simulink model "DSPB_MMSE"  (Simulink 8.1)
settings: Solver=VariableStepDiscrete  StartTime=0.0  StopTime=DSPB_MMSE_param.endTime  RelTol=1e-3
PreLoadFcn:
  | % Run the setup script when the model is opened
  | setup_DSPB_MMSE;
InitFcn:
  | % Run the setup script again just before the
  | % model is run, so that any updates made
  | % after opening are applied.
  | setup_DSPB_MMSE;
  | %% DSPBuilder Start
  | alt_dspbuilder_update_model(bdroot)
  | %% DSPBuilder End
StartFcn:
  | %% DSPBuilder Start
  | alt_dspbuilder_hdlimport_prepare_for_simulation(bdroot)
  | %% DSPBuilder End
undefined symbols (not defined in the file or in its folder): a, AdvDSPBDMemDisplay, dpoly, DSPB_MMSE_param, dspba, evalAionMaskParam, pow, primtype, UseDontCare, value, x, y
libraries: DSPBAPrim x213, DspbAdvFftLibrary x9, DSPBABase x5, simulink x3, DSPBAModelBus x3, DSPBAControl x1, DSPBAVectorUtil x1
(part 1 of 3)
Description:
  | DSP Builder Advanced Template for Template Design implementing Primitive Subsystems
settings Model: Creator=mjervis  LastModifiedBy=AliReza
settings DebuggingCC: InheritedTsInSrcMsg=none  IntegerOverflowMsg=none  FcnCallInpInsideContextMsg=EnableAllAsError  FrameProcessingCompatibilityMsg=error
settings GRTTargetCC: CodeReplacementLibrary=None  CPPClassGenCompliant=on

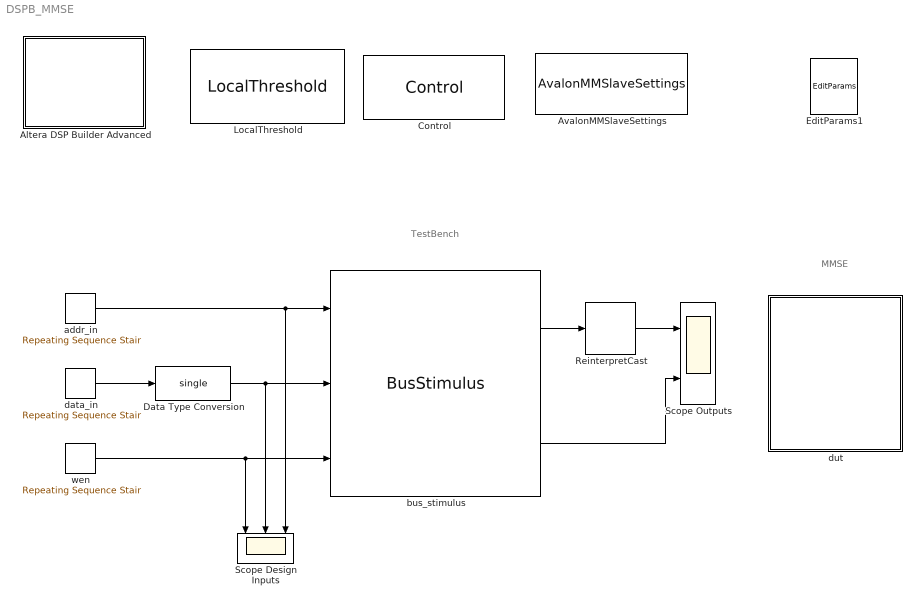
== system DSPB_MMSE ==
  note: MMSE
  note: TestBench
  Altera DSP Builder Advanced : Subsystem  mask(DSP Builder Advanced Blockset Ignored Block){}
      settings: OpenFcn=web('http://www.altera.com', '-new');
      mask Display: image(imread('intellogo.tif'));
  AvalonMMSlaveSettings : DSPBABase/AvalonMMSlaveSettings
  "Control " : DSPBABase/Control  generate=on  language=VHDL  destination=./rtl  make_full_path=off  path_is_relative=on  autotestbench=on  signaldepth=2  coveragetestbench=off  logs=off  spacewidth=2  spacenum=1  addrwidth=10  datawidth=16  dataendian=Big Endian  hierarchicalnames=on  ramThresholdBits=-1  distRamThresholdBits=-1  mlabThresholdBits=-1  hardMultiplierThresholdLuts=-1  version=20090407  errorOnChanMismatch=1  errorOnGPIOMismatch=0  importModelsimResults=0  cycleAccurate=off  reinterpretCastMult=off  paramFile=DSPB_MMSE_params.xml
  Data Type Conversion : DataTypeConversion  OutDataTypeStr=single
  EditParams1 : DSPBABase/EditParams  version=20090407
  LocalThreshold : DSPBABase/LocalThreshold  margin=0  delayRegOrRAMThresholdBits=-1  MediumDualMemThresholdBits=-1  LargeDualMemThresholdBits=0  hardMultiplierThresholdLuts=0  complexMultKaratsuba=off  version=0
  ReinterpretCast : DSPBAPrim/ReinterpretCast  primtype=reinterpret  nInputs=1  nOutputs=1  omode=single  otype=sfix(16)  scale=2^-15  rndmethod=Unbiased  factor=1  satmethod=Symmetric  shift_vec=[0 1 2 -1]  value=0  inPortNames=[' '; ' ';]  outPortNames=[' ']  dspbaimage=dspba_prim.jpg  text=fprintf('Reinterp\nCast', value);  style=Optimised  visibilities=8  floatPrecision=float32_m23  version=20120601
  Scope Outputs : Scope  NumInputPorts=2
      settings: YMin=-5~-5  YMax=5~5
  Scope Design Inputs : Scope  NumInputPorts=3
      settings: YMin=0~-0.05~-5  YMax=1~1~5
  addr_in : simulink/Sources/Repeating Sequence Stair  OutValues=DSPB_MMSE_IO.bus_addr_in  tsamp=1  OutMin=[]  OutMax=[]  OutDataTypeStr=Inherit: Inherit via back propagation  OutDataType=uint10  ConRadixGroup=Best Precision: Vector-wise  OutScaling=[]
  bus_stimulus : DSPBAModelBus/BusStimulus  SampleTime=-1  version=20140122  hasreaden=off
  data_in : simulink/Sources/Repeating Sequence Stair  OutValues=DSPB_MMSE_IO.bus_data_in  tsamp=1  OutMin=[]  OutMax=[]  OutDataTypeStr=double  OutputDataTypeScalingMode=double  OutDataType=fixdt(0,3)  ConRadixGroup=Best Precision: Vector-wise  OutScaling=[]
  dut : Subsystem
  wen : simulink/Sources/Repeating Sequence Stair  OutValues=DSPB_MMSE_IO.bus_wen  tsamp=1  OutMin=[]  OutMax=[]  OutDataTypeStr=fixdt('boolean')  OutputDataTypeScalingMode=Specify via dialog  OutDataType=fixdt('boolean')  ConRadixGroup=Best Precision: Vector-wise  OutScaling=[]
  wires:
  bus_stimulus/2 -> Scope Outputs/2
  addr_in/1 -> Scope Design Inputs/3, bus_stimulus/1
  wen/1 -> Scope Design Inputs/1, bus_stimulus/3
  data_in/1 -> Data Type Conversion/1
  Data Type Conversion/1 -> Scope Design Inputs/2, bus_stimulus/2
  bus_stimulus/1 -> ReinterpretCast/1
  ReinterpretCast/1 -> Scope Outputs/1

== system DSPB_MMSE/Altera DSP Builder Advanced ==

== system DSPB_MMSE/dut ==
  Device : DSPBABase/Device  family=Cyclone V  deviceMember=Stratix V GX  stratix4device=Stratix IV E  hardcopy4device=HardCopy IV E  stratix5device=Stratix V GX  device=AUTO  speed=-3  stratixSpeed=-5  stratix2Speed=-3  stratix3Speed=-2  stratix4gxSpeed=-2  stratix4gtSpeed=-1  cyclone2Speed=-6  cyclone3Speed=-7  arria2Speed=-4  cyclone4eSpeed=-8  stratix5Speed=-3  arria5Speed=-4  arriaSpeed=-6  cyclone3lsSpeed=-7  cyclone5Speed=-6  arria2gzSpeed=-3  nightFurySpeed=-2  ecp2Speed=-7  hardcopycompat=off  version=20140217  max10flashmode=off  max10nomeminit=off
  MMSE_TOP : Subsystem
  MM_in : Subsystem
  MM_out : Subsystem
  wires:
  MM_in/1(time_sample_valid) -> MMSE_TOP/1(valid)
  MM_in/2(time_sample_input) -> MMSE_TOP/2(sample_in)
  MMSE_TOP/1(_valid) -> MM_out/1(valid)
  MMSE_TOP/2(sample_out) -> MM_out/2(time_sample_output)

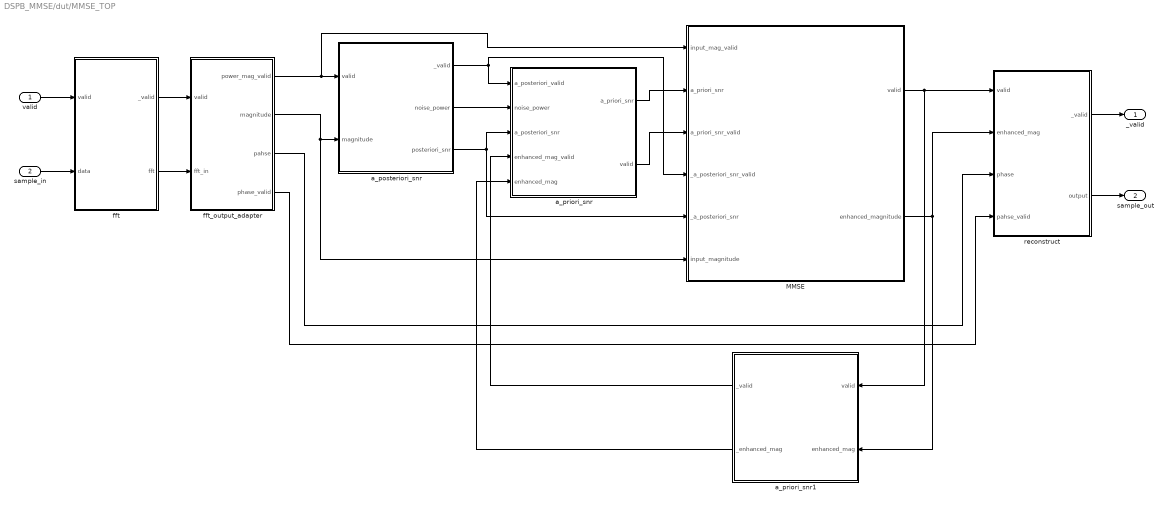
== system DSPB_MMSE/dut/MMSE_TOP ==
  valid : Inport
  sample_in : Inport  Port=2
  MMSE : Subsystem
  a_posteriori_snr : Subsystem
  a_priori_snr : Subsystem
  a_priori_snr1 : Subsystem
  fft : Subsystem
  fft_output_adapter : Subsystem
  reconstruct : Subsystem
  _valid : Outport
  sample_out : Outport  Port=2
  wires:
  fft_output_adapter/2(magnitude) -> MMSE/6(input_magnitude), a_posteriori_snr/2(magnitude)
  fft/1(_valid) -> fft_output_adapter/1(valid)
  fft/2(fft) -> fft_output_adapter/2(fft_in)
  fft_output_adapter/3(pahse) -> reconstruct/3(phase)
  fft_output_adapter/1(power_mag_valid) -> MMSE/1(input_mag_valid), a_posteriori_snr/1(valid)
  valid/1 -> fft/1(valid)
  sample_in/1 -> fft/2(data)
  fft_output_adapter/4(phase_valid) -> reconstruct/4(pahse_valid)
  reconstruct/1(_valid) -> _valid/1
  reconstruct/2(output) -> sample_out/1
  MMSE/1(valid) -> a_priori_snr1/1(valid), reconstruct/1(valid)
  MMSE/2(enhanced_magnitude) -> reconstruct/2(enhanced_mag), a_priori_snr1/2(enhanced_mag)
  a_priori_snr/1(a_priori_snr) -> MMSE/2(a_priori_snr)
  a_posteriori_snr/3(posteriori_snr) -> MMSE/5(_a_posteriori_snr), a_priori_snr/3(a_posteriori_snr)
  a_posteriori_snr/1(_valid) -> MMSE/4(_a_posteriori_snr_valid), a_priori_snr/1(a_posteriori_valid)
  a_posteriori_snr/2(noise_power) -> a_priori_snr/2(noise_power)
  a_priori_snr/2(valid) -> MMSE/3(a_priori_snr_valid)
  a_priori_snr1/2(_enhanced_mag) -> a_priori_snr/5(enhanced_mag)
  a_priori_snr1/1(_valid) -> a_priori_snr/4(enhanced_mag_valid)

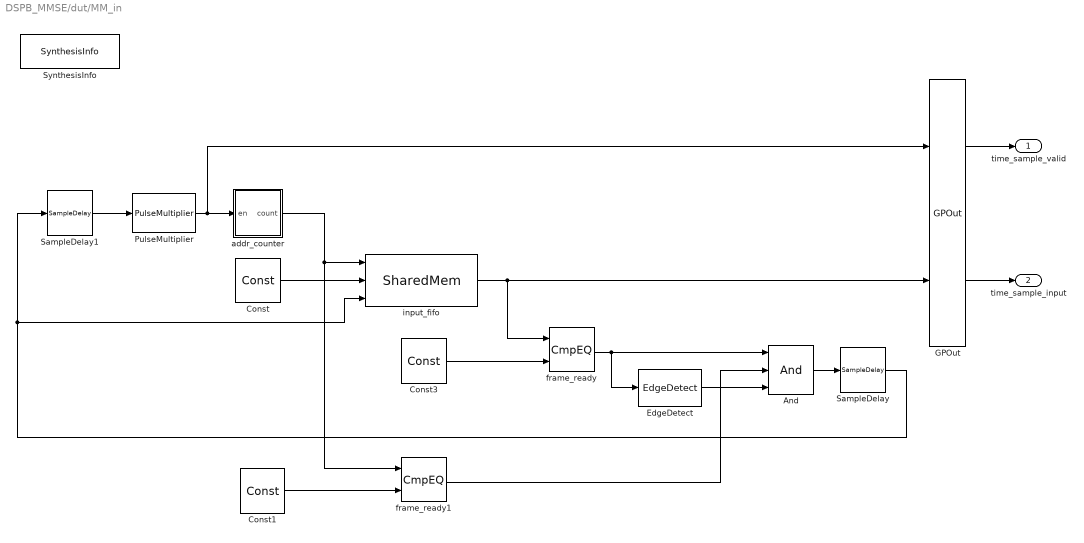
== system DSPB_MMSE/dut/MM_in ==
  And : DSPBAPrim/And  primtype=and  nInputs=3  nOutputs=1  omode=Inherit via internal rule  otype=sfix(16)  scale=2^-15  rndmethod=Unbiased  factor=1  satmethod=Symmetric  shift_vec=[0 1 2 -1]  value=0  inPortNames=[' '; ' '; ' '; ' '; ' '; ' '; ' '; ' '; ' '; ' '; ' '; ' '; ' '; ' '; ' '; ' '; ]  outPortNames=[' ']  dspbaimage=dspba_prim.jpg  text=fprintf('&');  style=Optimised  visibilities=8+2  version=20090407
  Const : DSPBAPrim/Const  primtype=const  nInputs=0  nOutputs=1  omode=single  otype=sfix(16)  scale=2^-15  rndmethod=Unbiased  factor=1  satmethod=Symmetric  shift_vec=[0 1 2 -1]  value=0  inPortNames=['+'; '+';]  outPortNames=[' ']  dspbaimage=dspba_prim.jpg  text=fprintf('%s', num2str(value));  style=Optimised  visibilities=8 + 1024  floatPrecision=float32_m23  version=20120820
  Const1 : DSPBAPrim/Const  primtype=const  nInputs=0  nOutputs=1  omode=Specify via dialog  otype=ufix(DSPB_MMSE_param.FS+1)  scale=2^-0  rndmethod=Unbiased  factor=1  satmethod=Symmetric  shift_vec=[0 1 2 -1]  value=0  inPortNames=['+'; '+';]  outPortNames=[' ']  dspbaimage=dspba_prim.jpg  text=fprintf('%s', num2str(value));  style=Optimised  visibilities=8 + 1024  floatPrecision=float32_m23  version=20120820
  Const3 : DSPBAPrim/Const  primtype=const  nInputs=0  nOutputs=1  omode=single  otype=sfix(16)  scale=2^-15  rndmethod=Unbiased  factor=1  satmethod=Symmetric  shift_vec=[0 1 2 -1]  value=1  inPortNames=['+'; '+';]  outPortNames=[' ']  dspbaimage=dspba_prim.jpg  text=fprintf('%s', num2str(value));  style=Optimised  visibilities=8 + 1024  floatPrecision=float32_m23  version=20120820
  EdgeDetect : DspbAdvFftLibrary/Common/EdgeDetect
  GPOut : DSPBAPrim/GPOut  primtype=gpout  nInputs=evalAionMaskParam(gcb,'value',1)  nOutputs=evalAionMaskParam(gcb,'value',1)  omode=Inherit via internal rule  otype=sfix(16)  scale=2^-15  rndmethod=Unbiased  factor=1  satmethod=Symmetric  shift_vec=[0 1 2 -1]  value=2  inPortNames=[' ' ' ' ' ' ' ' ' ' ' ' ' ' ' ' ' ' ' ' ' ' ' ' ' ' ' ' ' ' ' ' ' ' ' ' ' ' ' ' ' ' ' ' ' ' ' ' ' ' ' ' ' ' ' ' ' ' ' ' ' ' ' ' ' ' ' ' ' ']'  outPortNames=[' ' ' ' ' ' ' ' ' ' ' ' ' ' ' ' ' ' ' ' ' ' ' ' ' ' ' ' ' ' ' ' ' ' ' ' ' ' ' ' ' ' ' ' ' ' ' ' ' ' ' ' ' ' ' ' ' ' ' ' ' ' ' ' ' ' ' ' ' ']'  dspbaimage=dspba_prim.jpg  text=fprintf('GPOut');  style=Optimised  visibilities=1024  latencyCorrection=0  version=20090407
  PulseMultiplier : DspbAdvFftLibrary/Common/PulseMultiplier  N=DSPB_MMSE_param.FS
  SampleDelay : DSPBAPrim/SampleDelay  primtype=sampdelay  nInputs=1  nOutputs=1  omode=Inherit via internal rule  otype=sfix(16)  scale=2^-15  rndmethod=Unbiased  factor=1  satmethod=Symmetric  shift_vec=[0 1 2 -1]  value=3  inPortNames=[' '; ' ';]  outPortNames=[' ']  dspbaimage=dspba_prim.jpg  text=dpoly(1, eye(1,value+1), 'z')  style=Optimised  visibilities=8 + 1024 + 2^17 + 2^18  flexible=off  slackgroup=0  augmented=0  version=20090407  advOptions=[]
  SampleDelay1 : DSPBAPrim/SampleDelay  primtype=sampdelay  nInputs=1  nOutputs=1  omode=Inherit via internal rule  otype=sfix(16)  scale=2^-15  rndmethod=Unbiased  factor=1  satmethod=Symmetric  shift_vec=[0 1 2 -1]  value=1  inPortNames=[' '; ' ';]  outPortNames=[' ']  dspbaimage=dspba_prim.jpg  text=dpoly(1, eye(1,value+1), 'z')  style=Optimised  visibilities=8 + 1024 + 2^17 + 2^18  flexible=off  slackgroup=0  augmented=0  version=20090407  advOptions=[]
  SynthesisInfo : DSPBAPrim/SynthesisInfo  primtype=synthinfo  nInputs=0  nOutputs=0  omode=Inherit via internal rule  otype=sfix(16)  scale=2^-15  rndmethod=Truncate  factor=1  satmethod=Symmetric  shift_vec=[0 1 2 -1]  value=99  inPortNames=[' '; ' ';]  outPortNames=[' ']  dspbaimage=dspba_prim_ctrl.jpg  text=fprintf('Style=%s', style);  style=Scheduled  visibilities=2^17+2^18+2^19+2^20  constraintInUse=off  constraintRelation=>  constraintLimit=2  bitAccurate=off  version=20150220
  addr_counter : Subsystem
  frame_ready : DSPBAPrim/CmpEQ  primtype=cmpeq  nInputs=2  nOutputs=1  omode=boolean  otype=sfix(16)  scale=2^-15  rndmethod=Unbiased  factor=1  satmethod=Symmetric  shift_vec=[0 1 2 -1]  value=0  inPortNames=[' '; ' ';]  outPortNames=[' ']  dspbaimage=dspba_prim.jpg  text=fprintf('==');  style=Optimised  visibilities=0  advOptions=[]  version=20130117
  frame_ready1 : DSPBAPrim/CmpEQ  primtype=cmpeq  nInputs=2  nOutputs=1  omode=boolean  otype=sfix(16)  scale=2^-15  rndmethod=Unbiased  factor=1  satmethod=Symmetric  shift_vec=[0 1 2 -1]  value=0  inPortNames=[' '; ' ';]  outPortNames=[' ']  dspbaimage=dspba_prim.jpg  text=fprintf('==');  style=Optimised  visibilities=0  advOptions=[]  version=20130117
  input_fifo : DSPBAModelBus/SharedMem  mem_addr=0  mem_rwmode=Read/Write  mem_data=zeros(1,2^(DSPB_MMSE_param.FS)+1)  mem_init=on  mem_desc=input fifo  mem_mode=single  mem_type=sfix(16)  mem_scale=2^-8  SampleTime=-1  version=20090407
  time_sample_valid : Outport
  time_sample_input : Outport  Port=2
  wires:
  Const3/1 -> frame_ready/2
  And/1 -> SampleDelay/1
  SampleDelay/1 -> SampleDelay1/1, input_fifo/3
  addr_counter/1(count) -> input_fifo/1, frame_ready1/1
  SampleDelay1/1 -> PulseMultiplier/1
  frame_ready/1 -> EdgeDetect/1, And/1
  frame_ready1/1 -> And/2
  Const1/1 -> frame_ready1/2
  PulseMultiplier/1 -> GPOut/1, addr_counter/1(en)
  GPOut/2 -> time_sample_input/1
  EdgeDetect/1 -> And/3
  input_fifo/1 -> GPOut/2, frame_ready/1
  GPOut/1 -> time_sample_valid/1
  Const/1 -> input_fifo/2

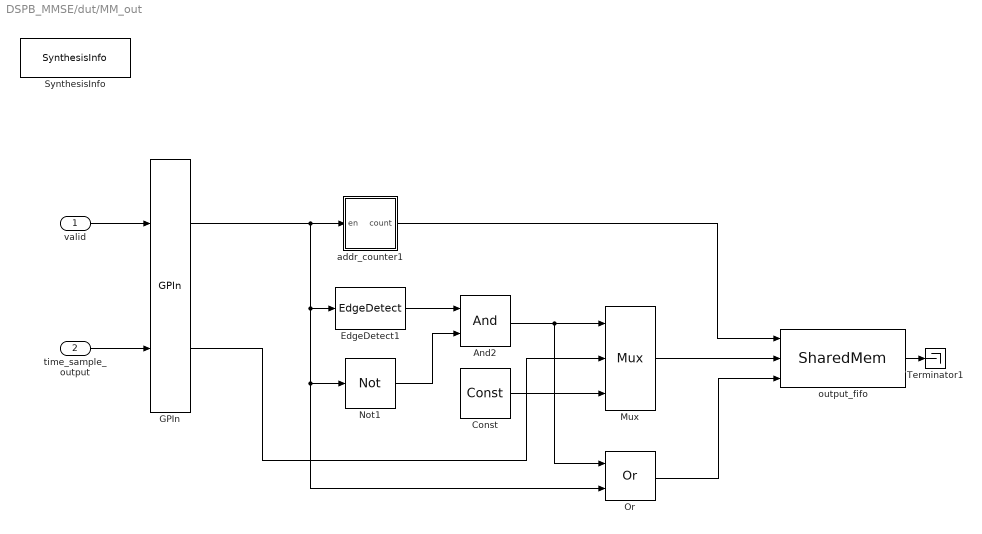
== system DSPB_MMSE/dut/MM_out ==
  valid : Inport
  time_sample_output : Inport  Port=2
  And2 : DSPBAPrim/And  primtype=and  nInputs=2  nOutputs=1  omode=Inherit via internal rule  otype=sfix(16)  scale=2^-15  rndmethod=Unbiased  factor=1  satmethod=Symmetric  shift_vec=[0 1 2 -1]  value=0  inPortNames=[' '; ' '; ' '; ' '; ' '; ' '; ' '; ' '; ' '; ' '; ' '; ' '; ' '; ' '; ' '; ' '; ]  outPortNames=[' ']  dspbaimage=dspba_prim.jpg  text=fprintf('&');  style=Optimised  visibilities=8+2  version=20090407
  Const : DSPBAPrim/Const  primtype=const  nInputs=0  nOutputs=1  omode=single  otype=sfix(16)  scale=2^-15  rndmethod=Unbiased  factor=1  satmethod=Symmetric  shift_vec=[0 1 2 -1]  value=1  inPortNames=['+'; '+';]  outPortNames=[' ']  dspbaimage=dspba_prim.jpg  text=fprintf('%s', num2str(value));  style=Optimised  visibilities=8 + 1024  floatPrecision=float32_m23  version=20120820
  EdgeDetect1 : DspbAdvFftLibrary/Common/EdgeDetect
  GPIn : DSPBAPrim/GPIn  primtype=gpin  nInputs=evalAionMaskParam(gcb,'value',1)  nOutputs=evalAionMaskParam(gcb,'value',1)  omode=Inherit via internal rule  otype=sfix(16)  scale=2^-15  rndmethod=Unbiased  factor=1  satmethod=Symmetric  shift_vec=[0 1 2 -1]  value=2  inPortNames=[' ' ' ' ' ' ' ' ' ' ' ' ' ' ' ' ' ' ' ' ' ' ' ' ' ' ' ' ' ' ' ' ' ' ' ' ' ' ' ' ' ' ' ' ' ' ' ' ' ' ' ' ' ' ' ' ' ' ' ' ' ' ' ' ' ' ' ' ' ']'  outPortNames=[' ' ' ' ' ' ' ' ' ' ' ' ' ' ' ' ' ' ' ' ' ' ' ' ' ' ' ' ' ' ' ' ' ' ' ' ' ' ' ' ' ' ' ' ' ' ' ' ' ' ' ' ' ' ' ' ' ' ' ' ' ' ' ' ' ' ' ' ' ']'  dspbaimage=dspba_prim.jpg  text=fprintf('GPIn');  style=Optimised  visibilities=1024  latencyCorrection=0  scheduleOrigin=on  version=20090407
  Mux : DSPBAPrim/Mux  primtype=mux  nInputs=evalAionMaskParam(gcb,'value',1)+1  nOutputs=1  omode=Inherit via internal rule  otype=sfix(16)  scale=2^-15  rndmethod=Unbiased  factor=1  satmethod=Symmetric  shift_vec=[0 1 2 -1]  value=2  inPortNames=['s '; 'd0'; 'd1'; 'd2'; 'd3'; 'd4'; 'd5'; 'd6'; 'd7'; 'd8'; 'd9';]  outPortNames=[' ']  dspbaimage=dspba_prim.jpg  text=fprintf('%s', primtype);  style=Optimised  visibilities=1032  version=20131025
  Not1 : DSPBAPrim/Not  primtype=not  nInputs=1  nOutputs=1  omode=Inherit via internal rule  otype=sfix(16)  scale=2^-15  rndmethod=Unbiased  factor=1  satmethod=Symmetric  shift_vec=[0 1 2 -1]  value=0  inPortNames=[' '; ' ';]  outPortNames=[' ']  dspbaimage=dspba_prim.jpg  text=fprintf('~');  style=Optimised  visibilities=8  version=20090407
  Or : DSPBAPrim/Or  primtype=or  nInputs=2  nOutputs=1  omode=Inherit via internal rule  otype=sfix(16)  scale=2^-15  rndmethod=Unbiased  factor=1  satmethod=Symmetric  shift_vec=[0 1 2 -1]  value=0  inPortNames=[' '; ' '; ' '; ' '; ' '; ' '; ' '; ' '; ' '; ' '; ' '; ' '; ' '; ' '; ' '; ' '; ]  outPortNames=[' ']  dspbaimage=dspba_prim.jpg  text=fprintf('|');  style=Optimised  visibilities=8+2  version=20090407
  SynthesisInfo : DSPBAPrim/SynthesisInfo  primtype=synthinfo  nInputs=0  nOutputs=0  omode=Inherit via internal rule  otype=sfix(16)  scale=2^-15  rndmethod=Truncate  factor=1  satmethod=Symmetric  shift_vec=[0 1 2 -1]  value=99  inPortNames=[' '; ' ';]  outPortNames=[' ']  dspbaimage=dspba_prim_ctrl.jpg  text=fprintf('Style=%s', style);  style=Scheduled  visibilities=2^17+2^18+2^19+2^20  constraintInUse=off  constraintRelation=>  constraintLimit=2  bitAccurate=off  version=20150220
  Terminator1 : Terminator
  addr_counter1 : Subsystem
  output_fifo : DSPBAModelBus/SharedMem  mem_addr=2^(DSPB_MMSE_param.FS)+1  mem_rwmode=Read/Write  mem_data=zeros(1,2^(DSPB_MMSE_param.FS)+1)  mem_init=on  mem_desc=output fifo  mem_mode=single  mem_type=sfix(16)  mem_scale=2^-8  SampleTime=-1  version=20090407
  wires:
  time_sample_output/1 -> GPIn/2
  valid/1 -> GPIn/1
  EdgeDetect1/1 -> And2/1
  Not1/1 -> And2/2
  Mux/1 -> output_fifo/2
  And2/1 -> Or/1, Mux/1
  output_fifo/1 -> Terminator1/1
  Const/1 -> Mux/3
  Or/1 -> output_fifo/3
  GPIn/1 -> Or/2, Not1/1, EdgeDetect1/1, addr_counter1/1(en)
  GPIn/2 -> Mux/2
  addr_counter1/1(count) -> output_fifo/1

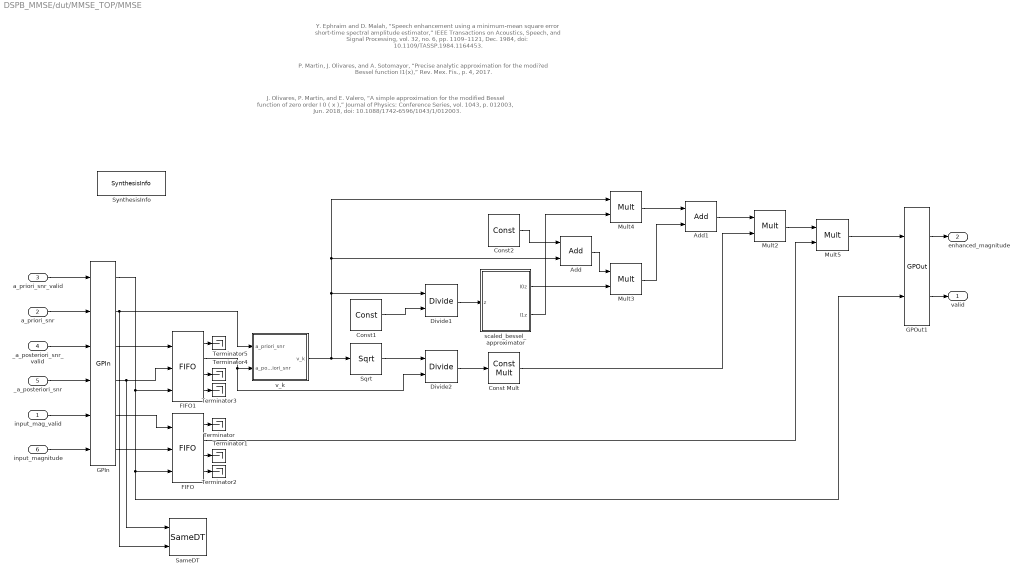
== system DSPB_MMSE/dut/MMSE_TOP/MMSE ==
  note: J. Olivares, P. Martin, and E. Valero, “A simple approximation for the modified Bessel function of zero order I 0 ( x ),”
      | Journal of Physics: Conference Series, vol. 1043, p. 012003, Jun. 2018, doi: 10.1088/1742-6596/1043/1/012003.
  note: P. Martin, J. Olivares, and A. Sotomayor, “Precise analytic approximation for the modi?ed Bessel function I1(x),” Rev. Mex. Fis., p. 4, 2017.
  note: Y. Ephraim and D. Malah, “Speech enhancement using a minimum-mean square error short-time spectral amplitude estimator,”
      |  IEEE Transactions on Acoustics, Speech, and Signal Processing, vol. 32, no. 6, pp. 1109–1121, Dec. 1984, doi: 10.1109/TASSP.1984.1164453.
  input_mag_valid : Inport
  a_priori_snr : Inport  Port=2
  a_priori_snr_valid : Inport  Port=3
  _a_posteriori_snr_valid : Inport  Port=4
  _a_posteriori_snr : Inport  Port=5
  input_magnitude : Inport  Port=6
  Add : DSPBAPrim/Add  primtype=add  nInputs=evalAionMaskParam(gcb,'value',1)  nOutputs=1  omode=Inherit via internal rule with word growth  otype=sfix(16)  scale=2^-15  rndmethod=Unbiased  factor=1  satmethod=Symmetric  shift_vec=[0 1 2 -1]  value=2  inPortNames=[' '; ' ';]  outPortNames=[' ']  dspbaimage=dspba_prim.jpg  text=fprintf('+');  style=Optimised  visibilities=1032+2^17+2^18+2^19  genFPC=off  floatRounding=correct  advOptions=[]  version=20130821
  Add1 : DSPBAPrim/Add  primtype=add  nInputs=evalAionMaskParam(gcb,'value',1)  nOutputs=1  omode=Inherit via internal rule with word growth  otype=sfix(16)  scale=2^-15  rndmethod=Unbiased  factor=1  satmethod=Symmetric  shift_vec=[0 1 2 -1]  value=2  inPortNames=[' '; ' ';]  outPortNames=[' ']  dspbaimage=dspba_prim.jpg  text=fprintf('+');  style=Optimised  visibilities=1032+2^17+2^18+2^19  genFPC=off  floatRounding=correct  advOptions=[]  version=20130821
  Const Mult : DSPBAPrim/Const Mult  primtype=constmult  nInputs=1  nOutputs=1  omode=Inherit via internal rule  otype=sfix(16)  scale=2^-15  rndmethod=Unbiased  factor=1  satmethod=Symmetric  shift_vec=[0 1 2 -1]  value=0.88622692545  inPortNames=[' '; ' ';]  outPortNames=[' ']  dspbaimage=dspba_prim.jpg  text=fprintf('cx');  style=Optimised  visibilities=8+2^10+2^17+2^18  floatRounding=correct  advOptions=[]  version=20140218
  Const1 : DSPBAPrim/Const  primtype=const  nInputs=0  nOutputs=1  omode=single  otype=sfix(16)  scale=2^-15  rndmethod=Unbiased  factor=1  satmethod=Symmetric  shift_vec=[0 1 2 -1]  value=2  inPortNames=['+'; '+';]  outPortNames=[' ']  dspbaimage=dspba_prim.jpg  text=fprintf('%s', num2str(value));  style=Optimised  visibilities=8 + 1024  floatPrecision=float32_m23  version=20120820
  Const2 : DSPBAPrim/Const  primtype=const  nInputs=0  nOutputs=1  omode=single  otype=sfix(16)  scale=2^-15  rndmethod=Unbiased  factor=1  satmethod=Symmetric  shift_vec=[0 1 2 -1]  value=1  inPortNames=['+'; '+';]  outPortNames=[' ']  dspbaimage=dspba_prim.jpg  text=fprintf('%s', num2str(value));  style=Optimised  visibilities=8 + 1024  floatPrecision=float32_m23  version=20120820
  Divide1 : DSPBAPrim/Divide  primtype=divide  nInputs=2  nOutputs=1  omode=Inherit via internal rule  otype=sfix(16)  scale=2^-15  rndmethod=Unbiased  factor=1  satmethod=Symmetric  shift_vec=[0 1 2 -1]  value=round([0:255]/17)  inPortNames=[' '; ' ';]  outPortNames=[' ']  dspbaimage=dspba_prim.jpg  text=fprintf('a\n----\nb');  style=Optimised  visibilities=8+2^17+2^18  floatRounding=correct  advOptions=[]  version=20130115
  Divide2 : DSPBAPrim/Divide  primtype=divide  nInputs=2  nOutputs=1  omode=Inherit via internal rule  otype=sfix(16)  scale=2^-15  rndmethod=Unbiased  factor=1  satmethod=Symmetric  shift_vec=[0 1 2 -1]  value=round([0:255]/17)  inPortNames=[' '; ' ';]  outPortNames=[' ']  dspbaimage=dspba_prim.jpg  text=fprintf('a\n----\nb');  style=Optimised  visibilities=8+2^17+2^18  floatRounding=correct  advOptions=[]  version=20130115
  FIFO : DSPBAPrim/FIFO  primtype=fifo  nInputs=3  nOutputs=4  omode=Inherit via internal rule  otype=sfix(16)  scale=2^-15  rndmethod=Unbiased  factor=1  satmethod=Symmetric  shift_vec=[0 1 2 -1]  value=[2^(DSPB_MMSE_param.FS-1) 1 2^(DSPB_MMSE_param.FS-1)]  inPortNames=['w'; 'd'; 'r'; 'f']  outPortNames=['v'; 'q'; 't'; 'f']  dspbaimage=dspba_prim.jpg  text=fprintf('fifo');  style=Optimised  visibilities=263168  version=20130808  user_sclr=off
  FIFO1 : DSPBAPrim/FIFO  primtype=fifo  nInputs=3  nOutputs=4  omode=Inherit via internal rule  otype=sfix(16)  scale=2^-15  rndmethod=Unbiased  factor=1  satmethod=Symmetric  shift_vec=[0 1 2 -1]  value=[2^(DSPB_MMSE_param.FS-1) 1 2^(DSPB_MMSE_param.FS-1)]  inPortNames=['w'; 'd'; 'r'; 'f']  outPortNames=['v'; 'q'; 't'; 'f']  dspbaimage=dspba_prim.jpg  text=fprintf('fifo');  style=Optimised  visibilities=263168  version=20130808  user_sclr=off
  GPIn : DSPBAPrim/GPIn  primtype=gpin  nInputs=evalAionMaskParam(gcb,'value',1)  nOutputs=evalAionMaskParam(gcb,'value',1)  omode=Inherit via internal rule  otype=sfix(16)  scale=2^-15  rndmethod=Unbiased  factor=1  satmethod=Symmetric  shift_vec=[0 1 2 -1]  value=6  inPortNames=[' ' ' ' ' ' ' ' ' ' ' ' ' ' ' ' ' ' ' ' ' ' ' ' ' ' ' ' ' ' ' ' ' ' ' ' ' ' ' ' ' ' ' ' ' ' ' ' ' ' ' ' ' ' ' ' ' ' ' ' ' ' ' ' ' ' ' ' ' ']'  outPortNames=[' ' ' ' ' ' ' ' ' ' ' ' ' ' ' ' ' ' ' ' ' ' ' ' ' ' ' ' ' ' ' ' ' ' ' ' ' ' ' ' ' ' ' ' ' ' ' ' ' ' ' ' ' ' ' ' ' ' ' ' ' ' ' ' ' ' ' ' ' ']'  dspbaimage=dspba_prim.jpg  text=fprintf('GPIn');  style=Optimised  visibilities=1024  latencyCorrection=0  scheduleOrigin=on  version=20090407
  GPOut1 : DSPBAPrim/GPOut  primtype=gpout  nInputs=evalAionMaskParam(gcb,'value',1)  nOutputs=evalAionMaskParam(gcb,'value',1)  omode=Inherit via internal rule  otype=sfix(16)  scale=2^-15  rndmethod=Unbiased  factor=1  satmethod=Symmetric  shift_vec=[0 1 2 -1]  value=2  inPortNames=[' ' ' ' ' ' ' ' ' ' ' ' ' ' ' ' ' ' ' ' ' ' ' ' ' ' ' ' ' ' ' ' ' ' ' ' ' ' ' ' ' ' ' ' ' ' ' ' ' ' ' ' ' ' ' ' ' ' ' ' ' ' ' ' ' ' ' ' ' ']'  outPortNames=[' ' ' ' ' ' ' ' ' ' ' ' ' ' ' ' ' ' ' ' ' ' ' ' ' ' ' ' ' ' ' ' ' ' ' ' ' ' ' ' ' ' ' ' ' ' ' ' ' ' ' ' ' ' ' ' ' ' ' ' ' ' ' ' ' ' ' ' ' ']'  dspbaimage=dspba_prim.jpg  text=fprintf('GPOut');  style=Optimised  visibilities=1024  latencyCorrection=0  version=20090407
  Mult{2..5} (4 alike) : DSPBAPrim/Mult  primtype=mult  nInputs=2  nOutputs=1  omode=Inherit via internal rule  otype=sfix(16)  scale=2^-15  rndmethod=Unbiased  factor=1  satmethod=Symmetric  shift_vec=[0 1 2 -1]  value=0  inPortNames=[' '; ' ';]  outPortNames=[' ']  dspbaimage=dspba_prim.jpg  text=fprintf('X');  style=Optimised  visibilities=8+2^18+2^19  floatPrecision=float32_m23  floatRounding=correct  advOptions=[]  version=20130115
  SameDT : DSPBAControl/SameDT
  Sqrt : DSPBAPrim/Sqrt  primtype=sqrtfunc  nInputs=1  nOutputs=1  omode=Inherit via internal rule  otype=sfix(16)  scale=2^-15  rndmethod=Unbiased  factor=1  satmethod=Symmetric  shift_vec=[0 1 2 -1]  value=round([0:255]/17)  inPortNames=[' '; ' ';]  outPortNames=[' ']  dspbaimage=dspba_prim_float.jpg  text=fprintf('sqrt(x)');  style=Optimised  visibilities=2^17  functionExpr=sqrt(x)  floatRounding=correct  advOptions=[]  version=20120730
  SynthesisInfo : DSPBAPrim/SynthesisInfo  primtype=synthinfo  nInputs=0  nOutputs=0  omode=Inherit via internal rule  otype=sfix(16)  scale=2^-15  rndmethod=Truncate  factor=1  satmethod=Symmetric  shift_vec=[0 1 2 -1]  value=99  inPortNames=[' '; ' ';]  outPortNames=[' ']  dspbaimage=dspba_prim_ctrl.jpg  text=fprintf('Style=%s', style);  style=Scheduled  visibilities=2^17+2^18+2^19+2^20  constraintInUse=off  constraintRelation=>  constraintLimit=2  bitAccurate=on  version=20150220
  Terminator{,1..5} (6 alike) : Terminator
  scaled_bessel_approximator : Subsystem
  v_k : Subsystem
  valid : Outport
  enhanced_magnitude : Outport  Port=2
  wires:
  a_priori_snr/1 -> GPIn/2
  _a_posteriori_snr/1 -> GPIn/4
  GPOut1/1 -> enhanced_magnitude/1
  GPOut1/2 -> valid/1
  Divide2/1 -> Const Mult/1
  Const1/1 -> Divide1/2
  Const Mult/1 -> Mult2/2
  Const2/1 -> Add/1
  Add/1 -> Mult3/1
  v_k/1(v_k) -> Divide1/1, Mult4/1, Add/2, Sqrt/1
  Mult3/1 -> Add1/2
  Mult4/1 -> Add1/1
  a_priori_snr_valid/1 -> GPIn/1
  input_magnitude/1 -> GPIn/6
  FIFO/1 -> Terminator/1
  FIFO/3 -> Terminator1/1
  FIFO/4 -> Terminator2/1
  input_mag_valid/1 -> GPIn/5
  Mult2/1 -> Mult5/1
  FIFO/2 -> Mult5/2
  Add1/1 -> Mult2/1
  scaled_bessel_approximator/1(I0z) -> Mult3/2
  scaled_bessel_approximator/2(I1z) -> Mult4/2
  Divide1/1 -> scaled_bessel_approximator/1(z)
  Sqrt/1 -> Divide2/1
  _a_posteriori_snr_valid/1 -> GPIn/3
  GPIn/3 -> FIFO1/1
  GPIn/4 -> SameDT/1, FIFO1/2
  GPIn/6 -> FIFO/2
  GPIn/5 -> FIFO/1
  GPIn/2 -> SameDT/2, v_k/1(a_priori_snr)
  FIFO1/2 -> Divide2/2, v_k/2(a_posteriori_snr)
  FIFO1/4 -> Terminator3/1
  FIFO1/3 -> Terminator4/1
  FIFO1/1 -> Terminator5/1
  Mult5/1 -> GPOut1/1
  GPIn/1 -> GPOut1/2, FIFO/3, FIFO1/3

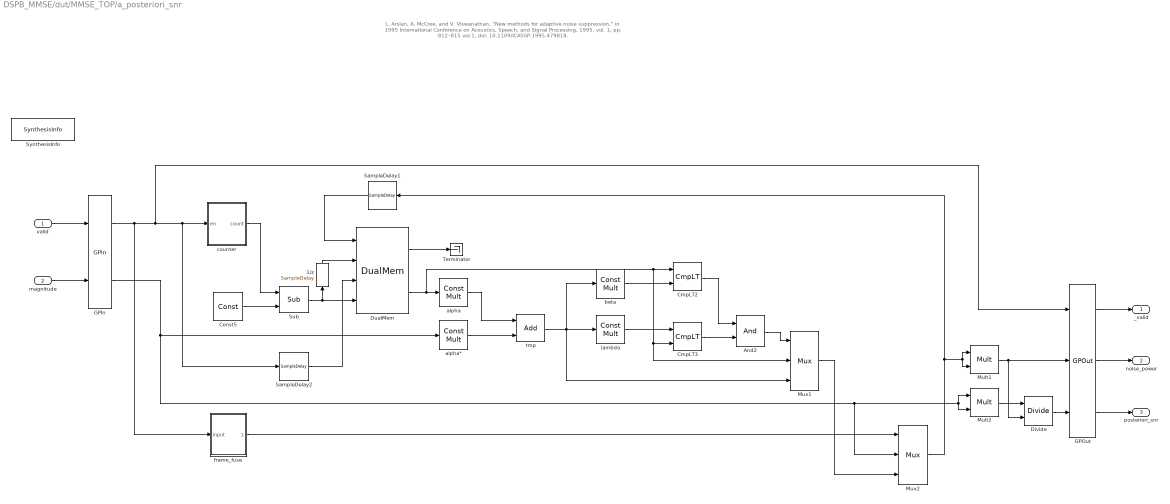
== system DSPB_MMSE/dut/MMSE_TOP/a_posteriori_snr ==
  note: L. Arslan, A. McCree, and V. Viswanathan, “New methods for adaptive noise suppression,”
      |  in 1995 International Conference on Acoustics, Speech, and Signal Processing, 1995,
      | vol. 1, pp. 812–815 vol.1, doi: 10.1109/ICASSP.1995.479818.
  valid : Inport
  magnitude : Inport  Port=2
  1/z : DSPBAPrim/SampleDelay  primtype=sampdelay  nInputs=1  nOutputs=1  omode=Inherit via internal rule  otype=sfix(16)  scale=2^-15  rndmethod=Unbiased  factor=1  satmethod=Symmetric  shift_vec=[0 1 2 -1]  value=6  inPortNames=[' '; ' ';]  outPortNames=[' ']  dspbaimage=dspba_prim.jpg  text=dpoly(1, eye(1,value+1), 'z')  style=Optimised  visibilities=8 + 1024 + 2^17 + 2^18  flexible=off  slackgroup=0  augmented=0  version=20090407  advOptions=[]
  And2 : DSPBAPrim/And  primtype=and  nInputs=2  nOutputs=1  omode=Inherit via internal rule  otype=sfix(16)  scale=2^-15  rndmethod=Unbiased  factor=1  satmethod=Symmetric  shift_vec=[0 1 2 -1]  value=0  inPortNames=[' '; ' '; ' '; ' '; ' '; ' '; ' '; ' '; ' '; ' '; ' '; ' '; ' '; ' '; ' '; ' '; ]  outPortNames=[' ']  dspbaimage=dspba_prim.jpg  text=fprintf('&');  style=Optimised  visibilities=8+2  version=20090407
  CmpLT2 : DSPBAPrim/CmpLT  primtype=cmplt  nInputs=2  nOutputs=1  omode=boolean  otype=sfix(16)  scale=2^-15  rndmethod=Unbiased  factor=1  satmethod=Symmetric  shift_vec=[0 1 2 -1]  value=0  inPortNames=['a'; 'b';]  outPortNames=[' ']  dspbaimage=dspba_prim.jpg  text=fprintf('a<b');  style=Optimised  visibilities=0  advOptions=[]  version=20130117
  CmpLT3 : DSPBAPrim/CmpLT  primtype=cmplt  nInputs=2  nOutputs=1  omode=boolean  otype=sfix(16)  scale=2^-15  rndmethod=Unbiased  factor=1  satmethod=Symmetric  shift_vec=[0 1 2 -1]  value=0  inPortNames=['a'; 'b';]  outPortNames=[' ']  dspbaimage=dspba_prim.jpg  text=fprintf('a<b');  style=Optimised  visibilities=0  advOptions=[]  version=20130117
  Const5 : DSPBAPrim/Const  primtype=const  nInputs=0  nOutputs=1  omode=Specify via dialog  otype=ufix(DSPB_MMSE_param.FS+1)  scale=2^-0  rndmethod=Unbiased  factor=1  satmethod=Symmetric  shift_vec=[0 1 2 -1]  value=1  inPortNames=['+'; '+';]  outPortNames=[' ']  dspbaimage=dspba_prim.jpg  text=fprintf('%s', num2str(value));  style=Optimised  visibilities=8 + 1024  floatPrecision=float32_m23  version=20120820
  Divide : DSPBAPrim/Divide  primtype=divide  nInputs=2  nOutputs=1  omode=Inherit via internal rule  otype=sfix(16)  scale=2^-15  rndmethod=Unbiased  factor=1  satmethod=Symmetric  shift_vec=[0 1 2 -1]  value=round([0:255]/17)  inPortNames=[' '; ' ';]  outPortNames=[' ']  dspbaimage=dspba_prim.jpg  text=fprintf('a\n----\nb');  style=Optimised  visibilities=8+2^17+2^18  floatRounding=correct  advOptions=[]  version=20130115
  DualMem : DSPBAPrim/DualMem  primtype=dualmem  nInputs=4  nOutputs=2  omode=single  otype=sfix(16)  scale=2^-15  rndmethod=Unbiased  factor=1  satmethod=Symmetric  shift_vec=[0 1 2 -1]  value=[zeros(2^DSPB_MMSE_param.FS, 1)]  inPortNames=['d1'; 'a1'; 'w1'; 'a2']  outPortNames=['q1'; 'q2']  dspbaimage=dspba_prim.jpg  text=fprintf('dmem%s',AdvDSPBDMemDisplay(UseDontCare));  style=Optimised  visibilities=8 + 1024 + 2^17 + 2^18  UseDontCare=on  TwinWritePorts=off  version=20141001
  GPIn : DSPBAPrim/GPIn  primtype=gpin  nInputs=evalAionMaskParam(gcb,'value',1)  nOutputs=evalAionMaskParam(gcb,'value',1)  omode=Inherit via internal rule  otype=sfix(16)  scale=2^-15  rndmethod=Unbiased  factor=1  satmethod=Symmetric  shift_vec=[0 1 2 -1]  value=2  inPortNames=[' ' ' ' ' ' ' ' ' ' ' ' ' ' ' ' ' ' ' ' ' ' ' ' ' ' ' ' ' ' ' ' ' ' ' ' ' ' ' ' ' ' ' ' ' ' ' ' ' ' ' ' ' ' ' ' ' ' ' ' ' ' ' ' ' ' ' ' ' ']'  outPortNames=[' ' ' ' ' ' ' ' ' ' ' ' ' ' ' ' ' ' ' ' ' ' ' ' ' ' ' ' ' ' ' ' ' ' ' ' ' ' ' ' ' ' ' ' ' ' ' ' ' ' ' ' ' ' ' ' ' ' ' ' ' ' ' ' ' ' ' ' ' ']'  dspbaimage=dspba_prim.jpg  text=fprintf('GPIn');  style=Optimised  visibilities=1024  latencyCorrection=0  scheduleOrigin=on  version=20090407
  GPOut : DSPBAPrim/GPOut  primtype=gpout  nInputs=evalAionMaskParam(gcb,'value',1)  nOutputs=evalAionMaskParam(gcb,'value',1)  omode=Inherit via internal rule  otype=sfix(16)  scale=2^-15  rndmethod=Unbiased  factor=1  satmethod=Symmetric  shift_vec=[0 1 2 -1]  value=3  inPortNames=[' ' ' ' ' ' ' ' ' ' ' ' ' ' ' ' ' ' ' ' ' ' ' ' ' ' ' ' ' ' ' ' ' ' ' ' ' ' ' ' ' ' ' ' ' ' ' ' ' ' ' ' ' ' ' ' ' ' ' ' ' ' ' ' ' ' ' ' ' ']'  outPortNames=[' ' ' ' ' ' ' ' ' ' ' ' ' ' ' ' ' ' ' ' ' ' ' ' ' ' ' ' ' ' ' ' ' ' ' ' ' ' ' ' ' ' ' ' ' ' ' ' ' ' ' ' ' ' ' ' ' ' ' ' ' ' ' ' ' ' ' ' ' ']'  dspbaimage=dspba_prim.jpg  text=fprintf('GPOut');  style=Optimised  visibilities=1024  latencyCorrection=0  version=20090407
  Mult1 : DSPBAPrim/Mult  primtype=mult  nInputs=2  nOutputs=1  omode=Inherit via internal rule  otype=sfix(16)  scale=2^-15  rndmethod=Unbiased  factor=1  satmethod=Symmetric  shift_vec=[0 1 2 -1]  value=0  inPortNames=[' '; ' ';]  outPortNames=[' ']  dspbaimage=dspba_prim.jpg  text=fprintf('X');  style=Optimised  visibilities=8+2^18+2^19  floatPrecision=float32_m23  floatRounding=correct  advOptions=[]  version=20130115
  Mult2 : DSPBAPrim/Mult  primtype=mult  nInputs=2  nOutputs=1  omode=Inherit via internal rule  otype=sfix(16)  scale=2^-15  rndmethod=Unbiased  factor=1  satmethod=Symmetric  shift_vec=[0 1 2 -1]  value=0  inPortNames=[' '; ' ';]  outPortNames=[' ']  dspbaimage=dspba_prim.jpg  text=fprintf('X');  style=Optimised  visibilities=8+2^18+2^19  floatPrecision=float32_m23  floatRounding=correct  advOptions=[]  version=20130115
  Mux1 : DSPBAPrim/Mux  primtype=mux  nInputs=evalAionMaskParam(gcb,'value',1)+1  nOutputs=1  omode=Inherit via internal rule  otype=sfix(16)  scale=2^-15  rndmethod=Unbiased  factor=1  satmethod=Symmetric  shift_vec=[0 1 2 -1]  value=2  inPortNames=['s '; 'd0'; 'd1'; 'd2'; 'd3'; 'd4'; 'd5'; 'd6'; 'd7'; 'd8'; 'd9';]  outPortNames=[' ']  dspbaimage=dspba_prim.jpg  text=fprintf('%s', primtype);  style=Optimised  visibilities=1032  version=20131025
  Mux2 : DSPBAPrim/Mux  primtype=mux  nInputs=evalAionMaskParam(gcb,'value',1)+1  nOutputs=1  omode=Inherit via internal rule  otype=sfix(16)  scale=2^-15  rndmethod=Unbiased  factor=1  satmethod=Symmetric  shift_vec=[0 1 2 -1]  value=2  inPortNames=['s '; 'd0'; 'd1'; 'd2'; 'd3'; 'd4'; 'd5'; 'd6'; 'd7'; 'd8'; 'd9';]  outPortNames=[' ']  dspbaimage=dspba_prim.jpg  text=fprintf('%s', primtype);  style=Optimised  visibilities=1032  version=20131025
  SampleDelay1 : DSPBAPrim/SampleDelay  primtype=sampdelay  nInputs=1  nOutputs=1  omode=Inherit via internal rule  otype=sfix(16)  scale=2^-15  rndmethod=Unbiased  factor=1  satmethod=Symmetric  shift_vec=[0 1 2 -1]  value=6  inPortNames=[' '; ' ';]  outPortNames=[' ']  dspbaimage=dspba_prim.jpg  text=dpoly(1, eye(1,value+1), 'z')  style=Optimised  visibilities=8 + 1024 + 2^17 + 2^18  flexible=off  slackgroup=0  augmented=0  version=20090407  advOptions=[]
  SampleDelay2 : DSPBAPrim/SampleDelay  primtype=sampdelay  nInputs=1  nOutputs=1  omode=Inherit via internal rule  otype=sfix(16)  scale=2^-15  rndmethod=Unbiased  factor=1  satmethod=Symmetric  shift_vec=[0 1 2 -1]  value=6  inPortNames=[' '; ' ';]  outPortNames=[' ']  dspbaimage=dspba_prim.jpg  text=dpoly(1, eye(1,value+1), 'z')  style=Optimised  visibilities=8 + 1024 + 2^17 + 2^18  flexible=off  slackgroup=0  augmented=0  version=20090407  advOptions=[]
  Sub : DSPBAPrim/Sub  primtype=sub  nInputs=2  nOutputs=1  omode=Specify via dialog  otype=ufix(DSPB_MMSE_param.FS+1)  scale=2^-0  rndmethod=Unbiased  factor=1  satmethod=Symmetric  shift_vec=[0 1 2 -1]  value=0  inPortNames=['+'; '-';]  outPortNames=[' ']  dspbaimage=dspba_prim.jpg  text=fprintf('-');  style=Optimised  visibilities=8+2^17+2^18  floatRounding=correct  advOptions=[]  version=20130115
  SynthesisInfo : DSPBAPrim/SynthesisInfo  primtype=synthinfo  nInputs=0  nOutputs=0  omode=Inherit via internal rule  otype=sfix(16)  scale=2^-15  rndmethod=Truncate  factor=1  satmethod=Symmetric  shift_vec=[0 1 2 -1]  value=99  inPortNames=[' '; ' ';]  outPortNames=[' ']  dspbaimage=dspba_prim_ctrl.jpg  text=fprintf('Style=%s', style);  style=Scheduled  visibilities=2^17+2^18+2^19+2^20  constraintInUse=off  constraintRelation=<  constraintLimit=10000  bitAccurate=on  version=20150220
  Terminator : Terminator
  alpha : DSPBAPrim/Const Mult  primtype=constmult  nInputs=1  nOutputs=1  omode=Inherit via internal rule  otype=sfix(16)  scale=2^-15  rndmethod=Unbiased  factor=1  satmethod=Symmetric  shift_vec=[0 1 2 -1]  value=0.9  inPortNames=[' '; ' ';]  outPortNames=[' ']  dspbaimage=dspba_prim.jpg  text=fprintf('cx');  style=Optimised  visibilities=8+2^10+2^17+2^18  floatRounding=correct  advOptions=[]  version=20140218
  alpha* : DSPBAPrim/Const Mult  primtype=constmult  nInputs=1  nOutputs=1  omode=Inherit via internal rule  otype=sfix(16)  scale=2^-15  rndmethod=Unbiased  factor=1  satmethod=Symmetric  shift_vec=[0 1 2 -1]  value=0.1  inPortNames=[' '; ' ';]  outPortNames=[' ']  dspbaimage=dspba_prim.jpg  text=fprintf('cx');  style=Optimised  visibilities=8+2^10+2^17+2^18  floatRounding=correct  advOptions=[]  version=20140218
  beta : DSPBAPrim/Const Mult  primtype=constmult  nInputs=1  nOutputs=1  omode=Inherit via internal rule  otype=sfix(16)  scale=2^-15  rndmethod=Unbiased  factor=1  satmethod=Symmetric  shift_vec=[0 1 2 -1]  value=1.2  inPortNames=[' '; ' ';]  outPortNames=[' ']  dspbaimage=dspba_prim.jpg  text=fprintf('cx');  style=Optimised  visibilities=8+2^10+2^17+2^18  floatRounding=correct  advOptions=[]  version=20140218
  counter : Subsystem
  frame_fuse : Subsystem
  lambda : DSPBAPrim/Const Mult  primtype=constmult  nInputs=1  nOutputs=1  omode=Inherit via internal rule  otype=sfix(16)  scale=2^-15  rndmethod=Unbiased  factor=1  satmethod=Symmetric  shift_vec=[0 1 2 -1]  value=0.85  inPortNames=[' '; ' ';]  outPortNames=[' ']  dspbaimage=dspba_prim.jpg  text=fprintf('cx');  style=Optimised  visibilities=8+2^10+2^17+2^18  floatRounding=correct  advOptions=[]  version=20140218
  tmp : DSPBAPrim/Add  primtype=add  nInputs=evalAionMaskParam(gcb,'value',1)  nOutputs=1  omode=Inherit via internal rule with word growth  otype=sfix(16)  scale=2^-15  rndmethod=Unbiased  factor=1  satmethod=Symmetric  shift_vec=[0 1 2 -1]  value=2  inPortNames=[' '; ' ';]  outPortNames=[' ']  dspbaimage=dspba_prim.jpg  text=fprintf('+');  style=Optimised  visibilities=1032+2^17+2^18+2^19  genFPC=off  floatRounding=correct  advOptions=[]  version=20130821
  _valid : Outport
  noise_power : Outport  Port=2
  posteriori_snr : Outport  Port=3
  wires:
  magnitude/1 -> GPIn/2
  valid/1 -> GPIn/1
  GPIn/1 -> frame_fuse/1(input), GPOut/1, counter/1(en), SampleDelay2/1
  counter/1(count) -> Sub/1
  Const5/1 -> Sub/2
  Sub/1 -> 1/z/1, DualMem/4
  GPIn/2 -> alpha*/1, Mux2/2, Mult2/2, Mult2/1
  DualMem/2 -> Mux1/2, CmpLT3/2, CmpLT2/1, alpha/1
  alpha*/1 -> tmp/2
  alpha/1 -> tmp/1
  tmp/1 -> beta/1, lambda/1, Mux1/3
  CmpLT2/1 -> And2/1
  CmpLT3/1 -> And2/2
  And2/1 -> Mux1/1
  beta/1 -> CmpLT2/2
  lambda/1 -> CmpLT3/1
  Mult1/1 -> Divide/2, GPOut/2
  SampleDelay1/1 -> DualMem/1
  1/z/1 -> DualMem/2
  SampleDelay2/1 -> DualMem/3
  GPOut/1 -> _valid/1
  GPOut/2 -> noise_power/1
  GPOut/3 -> posteriori_snr/1
  DualMem/1 -> Terminator/1
  frame_fuse/1(output) -> Mux2/1
  Mux1/1 -> Mux2/3
  Mux2/1 -> SampleDelay1/1, Mult1/1, Mult1/2
  Divide/1 -> GPOut/3
  Mult2/1 -> Divide/1

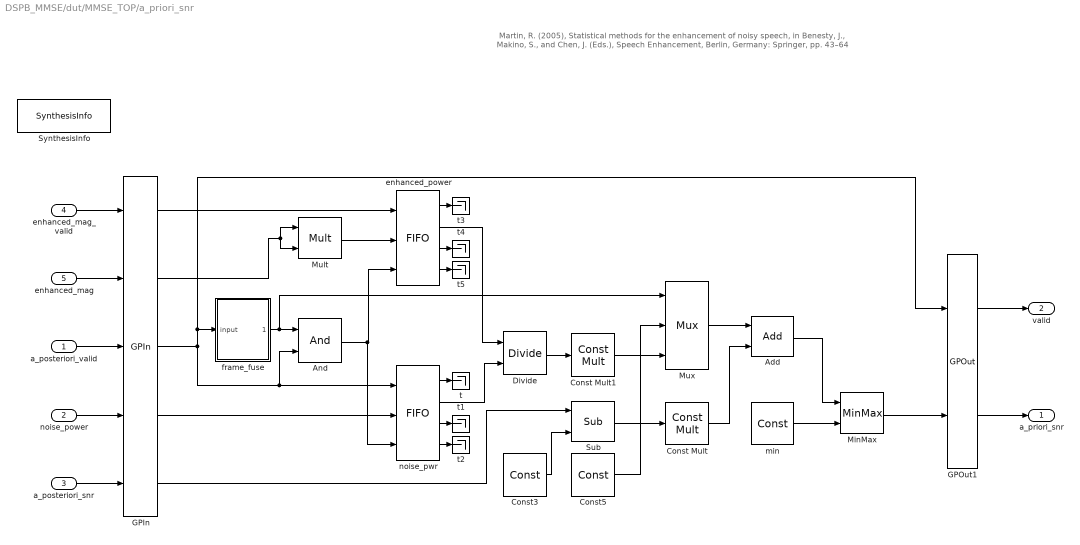
== system DSPB_MMSE/dut/MMSE_TOP/a_priori_snr ==
  note: Martin, R. (2005), Statistical methods for the enhancement of noisy speech,
      | in Benesty, J., Makino, S., and Chen, J. (Eds.), Speech Enhancement, Berlin, Germany:
      | Springer, pp. 43–64
  a_posteriori_valid : Inport
  noise_power : Inport  Port=2
  a_posteriori_snr : Inport  Port=3
  enhanced_mag_valid : Inport  Port=4
  enhanced_mag : Inport  Port=5
  Add : DSPBAPrim/Add  primtype=add  nInputs=evalAionMaskParam(gcb,'value',1)  nOutputs=1  omode=Inherit via internal rule with word growth  otype=sfix(16)  scale=2^-15  rndmethod=Unbiased  factor=1  satmethod=Symmetric  shift_vec=[0 1 2 -1]  value=2  inPortNames=[' '; ' ';]  outPortNames=[' ']  dspbaimage=dspba_prim.jpg  text=fprintf('+');  style=Optimised  visibilities=1032+2^17+2^18+2^19  genFPC=off  floatRounding=correct  advOptions=[]  version=20130821
  And : DSPBAPrim/And  primtype=and  nInputs=2  nOutputs=1  omode=Inherit via internal rule  otype=sfix(16)  scale=2^-15  rndmethod=Unbiased  factor=1  satmethod=Symmetric  shift_vec=[0 1 2 -1]  value=0  inPortNames=[' '; ' '; ' '; ' '; ' '; ' '; ' '; ' '; ' '; ' '; ' '; ' '; ' '; ' '; ' '; ' '; ]  outPortNames=[' ']  dspbaimage=dspba_prim.jpg  text=fprintf('&');  style=Optimised  visibilities=8+2  version=20090407
  Const Mult : DSPBAPrim/Const Mult  primtype=constmult  nInputs=1  nOutputs=1  omode=Inherit via internal rule  otype=sfix(16)  scale=2^-15  rndmethod=Unbiased  factor=1  satmethod=Symmetric  shift_vec=[0 1 2 -1]  value=0.02  inPortNames=[' '; ' ';]  outPortNames=[' ']  dspbaimage=dspba_prim.jpg  text=fprintf('cx');  style=Optimised  visibilities=8+2^10+2^17+2^18  floatRounding=correct  advOptions=[]  version=20140218
  Const Mult1 : DSPBAPrim/Const Mult  primtype=constmult  nInputs=1  nOutputs=1  omode=Inherit via internal rule  otype=sfix(16)  scale=2^-15  rndmethod=Unbiased  factor=1  satmethod=Symmetric  shift_vec=[0 1 2 -1]  value=0.98  inPortNames=[' '; ' ';]  outPortNames=[' ']  dspbaimage=dspba_prim.jpg  text=fprintf('cx');  style=Optimised  visibilities=8+2^10+2^17+2^18  floatRounding=correct  advOptions=[]  version=20140218
  Const3 : DSPBAPrim/Const  primtype=const  nInputs=0  nOutputs=1  omode=single  otype=sfix(16)  scale=2^-15  rndmethod=Unbiased  factor=1  satmethod=Symmetric  shift_vec=[0 1 2 -1]  value=1  inPortNames=['+'; '+';]  outPortNames=[' ']  dspbaimage=dspba_prim.jpg  text=fprintf('%s', num2str(value));  style=Optimised  visibilities=8 + 1024  floatPrecision=float32_m23  version=20120820
  Const5 : DSPBAPrim/Const  primtype=const  nInputs=0  nOutputs=1  omode=single  otype=sfix(16)  scale=2^-15  rndmethod=Unbiased  factor=1  satmethod=Symmetric  shift_vec=[0 1 2 -1]  value=0.98  inPortNames=['+'; '+';]  outPortNames=[' ']  dspbaimage=dspba_prim.jpg  text=fprintf('%s', num2str(value));  style=Optimised  visibilities=8 + 1024  floatPrecision=float32_m23  version=20120820
  Divide : DSPBAPrim/Divide  primtype=divide  nInputs=2  nOutputs=1  omode=Inherit via internal rule  otype=sfix(16)  scale=2^-15  rndmethod=Unbiased  factor=1  satmethod=Symmetric  shift_vec=[0 1 2 -1]  value=round([0:255]/17)  inPortNames=[' '; ' ';]  outPortNames=[' ']  dspbaimage=dspba_prim.jpg  text=fprintf('a\n----\nb');  style=Optimised  visibilities=8+2^17+2^18  floatRounding=correct  advOptions=[]  version=20130115
  GPIn : DSPBAPrim/GPIn  primtype=gpin  nInputs=evalAionMaskParam(gcb,'value',1)  nOutputs=evalAionMaskParam(gcb,'value',1)  omode=Inherit via internal rule  otype=sfix(16)  scale=2^-15  rndmethod=Unbiased  factor=1  satmethod=Symmetric  shift_vec=[0 1 2 -1]  value=5  inPortNames=[' ' ' ' ' ' ' ' ' ' ' ' ' ' ' ' ' ' ' ' ' ' ' ' ' ' ' ' ' ' ' ' ' ' ' ' ' ' ' ' ' ' ' ' ' ' ' ' ' ' ' ' ' ' ' ' ' ' ' ' ' ' ' ' ' ' ' ' ' ']'  outPortNames=[' ' ' ' ' ' ' ' ' ' ' ' ' ' ' ' ' ' ' ' ' ' ' ' ' ' ' ' ' ' ' ' ' ' ' ' ' ' ' ' ' ' ' ' ' ' ' ' ' ' ' ' ' ' ' ' ' ' ' ' ' ' ' ' ' ' ' ' ' ']'  dspbaimage=dspba_prim.jpg  text=fprintf('GPIn');  style=Optimised  visibilities=1024  latencyCorrection=0  scheduleOrigin=on  version=20090407
  GPOut1 : DSPBAPrim/GPOut  primtype=gpout  nInputs=evalAionMaskParam(gcb,'value',1)  nOutputs=evalAionMaskParam(gcb,'value',1)  omode=Inherit via internal rule  otype=sfix(16)  scale=2^-15  rndmethod=Unbiased  factor=1  satmethod=Symmetric  shift_vec=[0 1 2 -1]  value=2  inPortNames=[' ' ' ' ' ' ' ' ' ' ' ' ' ' ' ' ' ' ' ' ' ' ' ' ' ' ' ' ' ' ' ' ' ' ' ' ' ' ' ' ' ' ' ' ' ' ' ' ' ' ' ' ' ' ' ' ' ' ' ' ' ' ' ' ' ' ' ' ' ']'  outPortNames=[' ' ' ' ' ' ' ' ' ' ' ' ' ' ' ' ' ' ' ' ' ' ' ' ' ' ' ' ' ' ' ' ' ' ' ' ' ' ' ' ' ' ' ' ' ' ' ' ' ' ' ' ' ' ' ' ' ' ' ' ' ' ' ' ' ' ' ' ' ']'  dspbaimage=dspba_prim.jpg  text=fprintf('GPOut');  style=Optimised  visibilities=1024  latencyCorrection=0  version=20090407
  MinMax : DSPBAPrim/MinMax  primtype=minmaxfunc  nInputs=2  nOutputs=1  omode=Inherit via internal rule  otype=sfix(16)  scale=2^-15  rndmethod=Unbiased  factor=1  satmethod=Symmetric  shift_vec=[0 1 2 -1]  value=0  inPortNames=[' '; ' ';]  outPortNames=[' ']  dspbaimage=dspba_prim.jpg  text=disp('min');  style=Optimised  visibilities=8+2^17  functionExpr=max  advOptions=[]  version=20121130
  Mult : DSPBAPrim/Mult  primtype=mult  nInputs=2  nOutputs=1  omode=Inherit via internal rule  otype=dspba.namedVPFloat('single')  scale=2^-0  rndmethod=Unbiased  factor=1  satmethod=Symmetric  shift_vec=[0 1 2 -1]  value=0  inPortNames=[' '; ' ';]  outPortNames=[' ']  dspbaimage=dspba_prim.jpg  text=fprintf('X');  style=Optimised  visibilities=8+2^18+2^19  floatPrecision=float32_m23  floatRounding=correct  advOptions=[]  version=20130115
  Mux : DSPBAPrim/Mux  primtype=mux  nInputs=evalAionMaskParam(gcb,'value',1)+1  nOutputs=1  omode=Inherit via internal rule  otype=dspba.namedVPFloat('single')  scale=2^-0  rndmethod=Unbiased  factor=1  satmethod=Symmetric  shift_vec=[0 1 2 -1]  value=2  inPortNames=['s '; 'd0'; 'd1'; 'd2'; 'd3'; 'd4'; 'd5'; 'd6'; 'd7'; 'd8'; 'd9';]  outPortNames=[' ']  dspbaimage=dspba_prim.jpg  text=fprintf('%s', primtype);  style=Optimised  visibilities=1032  version=20131025
  Sub : DSPBAPrim/Sub  primtype=sub  nInputs=2  nOutputs=1  omode=Inherit via internal rule with word growth  otype=sfix(16)  scale=2^-15  rndmethod=Unbiased  factor=1  satmethod=Symmetric  shift_vec=[0 1 2 -1]  value=0  inPortNames=['+'; '-';]  outPortNames=[' ']  dspbaimage=dspba_prim.jpg  text=fprintf('-');  style=Optimised  visibilities=8+2^17+2^18  floatRounding=correct  advOptions=[]  version=20130115
  SynthesisInfo : DSPBAPrim/SynthesisInfo  primtype=synthinfo  nInputs=0  nOutputs=0  omode=Inherit via internal rule  otype=sfix(16)  scale=2^-15  rndmethod=Truncate  factor=1  satmethod=Symmetric  shift_vec=[0 1 2 -1]  value=99  inPortNames=[' '; ' ';]  outPortNames=[' ']  dspbaimage=dspba_prim_ctrl.jpg  text=fprintf('Style=%s', style);  style=Scheduled  visibilities=2^17+2^18+2^19+2^20  constraintInUse=off  constraintRelation=>  constraintLimit=2  bitAccurate=on  version=20150220
  enhanced_power : DSPBAPrim/FIFO  primtype=fifo  nInputs=3  nOutputs=4  omode=Inherit via internal rule  otype=sfix(16)  scale=2^-15  rndmethod=Unbiased  factor=1  satmethod=Symmetric  shift_vec=[0 1 2 -1]  value=[2^(DSPB_MMSE_param.FS-1) 1 2^(DSPB_MMSE_param.FS-1)]  inPortNames=['w'; 'd'; 'r'; 'f']  outPortNames=['v'; 'q'; 't'; 'f']  dspbaimage=dspba_prim.jpg  text=fprintf('fifo');  style=Optimised  visibilities=263168  version=20130808  user_sclr=off
  frame_fuse : Subsystem
  min : DSPBAPrim/Const  primtype=const  nInputs=0  nOutputs=1  omode=single  otype=sfix(16)  scale=2^-15  rndmethod=Unbiased  factor=1  satmethod=Symmetric  shift_vec=[0 1 2 -1]  value=0.032  inPortNames=['+'; '+';]  outPortNames=[' ']  dspbaimage=dspba_prim.jpg  text=fprintf('%s', num2str(value));  style=Optimised  visibilities=8 + 1024  floatPrecision=float32_m23  version=20120820
  noise_pwr : DSPBAPrim/FIFO  primtype=fifo  nInputs=3  nOutputs=4  omode=Inherit via internal rule  otype=sfix(16)  scale=2^-15  rndmethod=Unbiased  factor=1  satmethod=Symmetric  shift_vec=[0 1 2 -1]  value=[2^(DSPB_MMSE_param.FS-1)+1 1 2^(DSPB_MMSE_param.FS-1)+1]  inPortNames=['w'; 'd'; 'r'; 'f']  outPortNames=['v'; 'q'; 't'; 'f']  dspbaimage=dspba_prim.jpg  text=fprintf('fifo');  style=Optimised  visibilities=263168  version=20130808  user_sclr=off
  t{,1..5} (6 alike) : Terminator
  a_priori_snr : Outport
  valid : Outport  Port=2
  wires:
  Const3/1 -> Sub/2
  Sub/1 -> Const Mult/1
  min/1 -> MinMax/2
  Const5/1 -> Mux/2
  Mux/1 -> Add/1
  Const Mult/1 -> Add/2
  Const Mult1/1 -> Mux/3
  GPOut1/2 -> a_priori_snr/1
  MinMax/1 -> GPOut1/2
  Add/1 -> MinMax/1
  enhanced_mag_valid/1 -> GPIn/1
  enhanced_mag/1 -> GPIn/2
  GPOut1/1 -> valid/1
  a_posteriori_valid/1 -> GPIn/3
  a_posteriori_snr/1 -> GPIn/5
  noise_power/1 -> GPIn/4
  Divide/1 -> Const Mult1/1
  GPIn/5 -> Sub/1
  GPIn/3 -> And/2, noise_pwr/1, GPOut1/1, frame_fuse/1(input)
  GPIn/4 -> noise_pwr/2
  GPIn/2 -> Mult/1, Mult/2
  GPIn/1 -> enhanced_power/1
  enhanced_power/2 -> Divide/1
  noise_pwr/2 -> Divide/2
  noise_pwr/3 -> t1/1
  noise_pwr/1 -> t/1
  noise_pwr/4 -> t2/1
  enhanced_power/1 -> t3/1
  enhanced_power/3 -> t4/1
  enhanced_power/4 -> t5/1
  frame_fuse/1(output) -> Mux/1, And/1
  And/1 -> noise_pwr/3, enhanced_power/3
  Mult/1 -> enhanced_power/2

== system DSPB_MMSE/dut/MMSE_TOP/a_priori_snr1 ==
  valid : Inport
  enhanced_mag : Inport  Port=2
  GPIn : DSPBAPrim/GPIn  primtype=gpin  nInputs=evalAionMaskParam(gcb,'value',1)  nOutputs=evalAionMaskParam(gcb,'value',1)  omode=Inherit via internal rule  otype=sfix(16)  scale=2^-15  rndmethod=Unbiased  factor=1  satmethod=Symmetric  shift_vec=[0 1 2 -1]  value=2  inPortNames=[' ' ' ' ' ' ' ' ' ' ' ' ' ' ' ' ' ' ' ' ' ' ' ' ' ' ' ' ' ' ' ' ' ' ' ' ' ' ' ' ' ' ' ' ' ' ' ' ' ' ' ' ' ' ' ' ' ' ' ' ' ' ' ' ' ' ' ' ' ']'  outPortNames=[' ' ' ' ' ' ' ' ' ' ' ' ' ' ' ' ' ' ' ' ' ' ' ' ' ' ' ' ' ' ' ' ' ' ' ' ' ' ' ' ' ' ' ' ' ' ' ' ' ' ' ' ' ' ' ' ' ' ' ' ' ' ' ' ' ' ' ' ' ']'  dspbaimage=dspba_prim.jpg  text=fprintf('GPIn');  style=Optimised  visibilities=1024  latencyCorrection=0  scheduleOrigin=on  version=20090407
  GPOut1 : DSPBAPrim/GPOut  primtype=gpout  nInputs=evalAionMaskParam(gcb,'value',1)  nOutputs=evalAionMaskParam(gcb,'value',1)  omode=Inherit via internal rule  otype=sfix(16)  scale=2^-15  rndmethod=Unbiased  factor=1  satmethod=Symmetric  shift_vec=[0 1 2 -1]  value=2  inPortNames=[' ' ' ' ' ' ' ' ' ' ' ' ' ' ' ' ' ' ' ' ' ' ' ' ' ' ' ' ' ' ' ' ' ' ' ' ' ' ' ' ' ' ' ' ' ' ' ' ' ' ' ' ' ' ' ' ' ' ' ' ' ' ' ' ' ' ' ' ' ']'  outPortNames=[' ' ' ' ' ' ' ' ' ' ' ' ' ' ' ' ' ' ' ' ' ' ' ' ' ' ' ' ' ' ' ' ' ' ' ' ' ' ' ' ' ' ' ' ' ' ' ' ' ' ' ' ' ' ' ' ' ' ' ' ' ' ' ' ' ' ' ' ' ']'  dspbaimage=dspba_prim.jpg  text=fprintf('GPOut');  style=Optimised  visibilities=1024  latencyCorrection=0  version=20090407
  SynthesisInfo : DSPBAPrim/SynthesisInfo  primtype=synthinfo  nInputs=0  nOutputs=0  omode=Inherit via internal rule  otype=sfix(16)  scale=2^-15  rndmethod=Truncate  factor=1  satmethod=Symmetric  shift_vec=[0 1 2 -1]  value=99  inPortNames=[' '; ' ';]  outPortNames=[' ']  dspbaimage=dspba_prim_ctrl.jpg  text=fprintf('Style=%s', style);  style=Scheduled  visibilities=2^17+2^18+2^19+2^20  constraintInUse=off  constraintRelation=>  constraintLimit=2  bitAccurate=on  version=20150220
  enhanced_power : DSPBAPrim/FIFO  primtype=fifo  nInputs=3  nOutputs=4  omode=Inherit via internal rule  otype=sfix(16)  scale=2^-15  rndmethod=Unbiased  factor=1  satmethod=Symmetric  shift_vec=[0 1 2 -1]  value=[4 1 4]  inPortNames=['w'; 'd'; 'r'; 'f']  outPortNames=['v'; 'q'; 't'; 'f']  dspbaimage=dspba_prim.jpg  text=fprintf('fifo');  style=Optimised  visibilities=263168  version=20130808  user_sclr=off
  t4 : Terminator
  t5 : Terminator
  _valid : Outport
  _enhanced_mag : Outport  Port=2
  wires:
  GPOut1/2 -> _enhanced_mag/1
  valid/1 -> GPIn/1
  GPOut1/1 -> _valid/1
  enhanced_power/1 -> enhanced_power/3, GPOut1/1
  enhanced_power/3 -> t4/1
  enhanced_power/4 -> t5/1
  enhanced_mag/1 -> GPIn/2
  GPIn/1 -> enhanced_power/1
  GPIn/2 -> enhanced_power/2
  enhanced_power/2 -> GPOut1/2
